simulink model "monitor"  (R2019b)
settings: Solver=FixedStepAuto  StartTime=0.0  StopTime=inf  FixedStep=0.01  RelTol=1e-3
undefined symbols (not defined in the file or in its folder): Command, f, serial
libraries: instrumentlib x5, simulink x3
settings Model: EnablePacing=on  Creator=Quinn  LastModifiedBy=Quinn

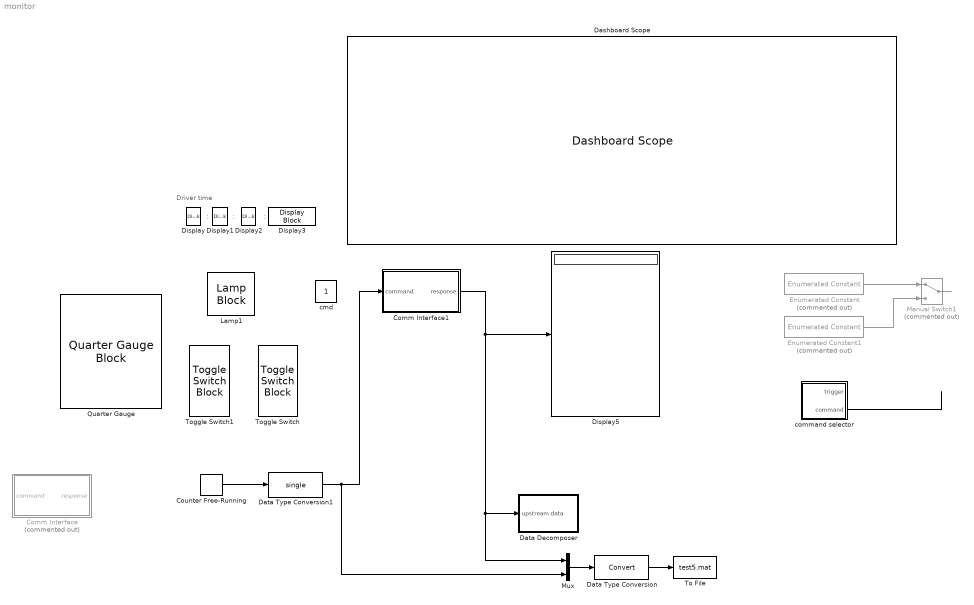
== system monitor ==
  note: :
  note: Driver time
  note: :
  note: :
  Comm Interface : Subsystem  Commented=on
  Comm Interface1 : Subsystem
  Counter Free-Running : simulink/Sources/Counter Free-Running  NumBits=16  tsamp=-1
  Dashboard Scope : DashboardScope  TimeSpan=30  Ymin=-0.5  Ymax=130
  Data Decomposer : Subsystem
  Data Type Conversion : DataTypeConversion
  Data Type Conversion1 : DataTypeConversion  OutDataTypeStr=single
  Display{,1..3} (4 alike) : DisplayBlock  LabelPosition=Hide  Format=short  Transparency=1  Opacity=0
  Display5 : Display
  Enumerated Constant : simulink/Sources/Enumerated Constant  Commented=on  OutDataTypeStr=Enum: Command  Value=Command.BX  SampleTime=inf
      settings: SourceProductName=Simulink
  Enumerated Constant1 : simulink/Sources/Enumerated Constant  Commented=on  OutDataTypeStr=Enum: Command  Value=Command.STOP  SampleTime=inf
      settings: SourceProductName=Simulink
  Lamp1 : LampBlock  LabelPosition=Bottom
  Manual Switch1 : ManualSwitch  Commented=on
  Mux : Mux  Inputs=2
  Quarter Gauge : QuarterGaugeBlock  ScaleMax=5
  To File : ToFile  Filename=test5.mat  MatrixName=data
  Toggle Switch : ToggleSwitchBlock  LabelPosition=Hide
      settings: Values={{'Log OFF', 'Log ON'}, [0 1]}
  Toggle Switch1 : ToggleSwitchBlock  LabelPosition=Hide
      settings: Values={{'PWR OFF', 'PWR ON'}, [0 1]}
  cmd : Constant  OutDataTypeStr=single
  command selector : Subsystem
  wires:
  Enumerated Constant/1 -> Manual Switch1/1
  Manual Switch1/1 -> ?
  Enumerated Constant1/1 -> Manual Switch1/2
  command selector/2(command) -> ?
  Comm Interface1/1(response) -> Mux/1, Data Decomposer/1(upstream data), Display5/1
  Data Type Conversion/1 -> To File/1
  Counter Free-Running/1 -> Data Type Conversion1/1
  Data Type Conversion1/1 -> Mux/2, Comm Interface1/1(command)
  Mux/1 -> Data Type Conversion/1

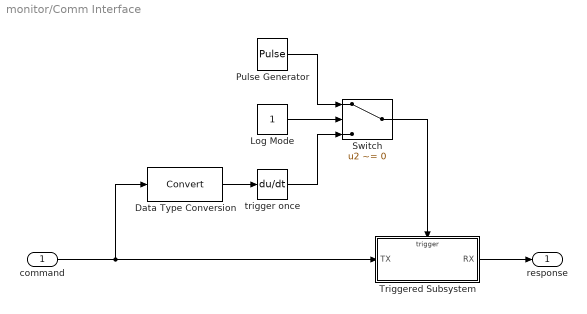
== system monitor/Comm Interface ==
  command : Inport
  Data Type Conversion : DataTypeConversion
  Log Mode : Constant
  Pulse Generator : DiscretePulseGenerator  SampleTime=0.01
  Switch : Switch  Criteria=u2 ~= 0
  Triggered Subsystem : Subsystem  Priority=1  TreatAsAtomicUnit=on
  trigger once : Derivative
  response : Outport
  wires:
  Triggered Subsystem/1(RX) -> response/1
  Log Mode/1 -> Switch/2
  Switch/1 -> Triggered Subsystem/Trigger
  Pulse Generator/1 -> Switch/1
  command/1 -> Triggered Subsystem/1(TX), Data Type Conversion/1
  trigger once/1 -> Switch/3
  Data Type Conversion/1 -> trigger once/1

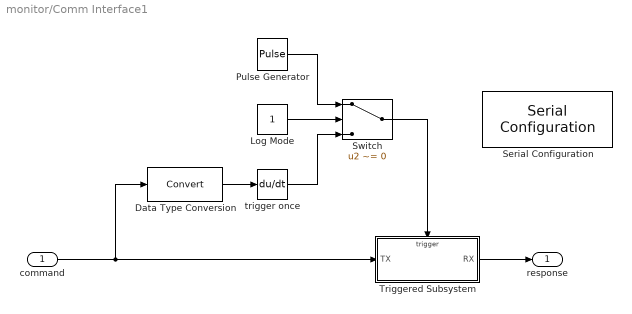
== system monitor/Comm Interface1 ==
  command : Inport
  Data Type Conversion : DataTypeConversion
  Log Mode : Constant
  Pulse Generator : DiscretePulseGenerator  SampleTime=0.01
  Serial Configuration : instrumentlib/Serial Configuration  Priority=-200000  ComPortMenu=COM5  ComPort=COM5  ObjConstructor=serial('COM5');  BaudRate=5e6  DataBits=8  Parity=none  StopBits=1  FlowControl=none  Timeout=1  ByteOrder=LittleEndian
  Switch : Switch  Criteria=u2 ~= 0
  Triggered Subsystem : Subsystem  Priority=1  TreatAsAtomicUnit=on
  trigger once : Derivative
  response : Outport
  wires:
  Data Type Conversion/1 -> trigger once/1
  trigger once/1 -> Switch/3
  command/1 -> Data Type Conversion/1, Triggered Subsystem/1(TX)
  Pulse Generator/1 -> Switch/1
  Switch/1 -> Triggered Subsystem/Trigger
  Log Mode/1 -> Switch/2
  Triggered Subsystem/1(RX) -> response/1

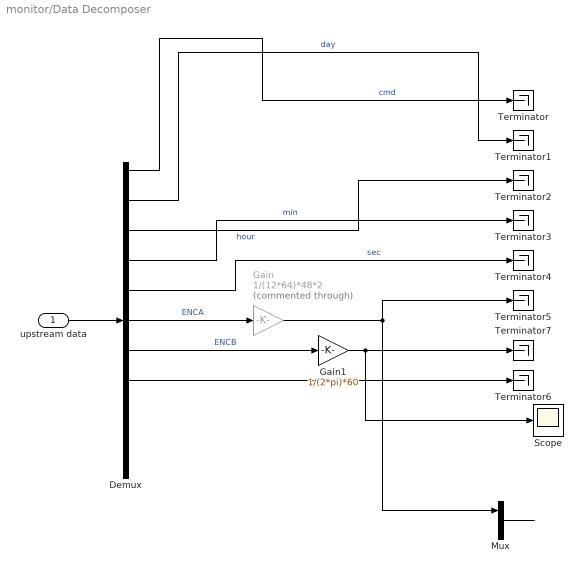
== system monitor/Data Decomposer ==
  upstream data : Inport
  Demux : Demux  Outputs=11
  Gain : Gain  Commented=through  Gain=1/(12*64)*48*2
  Gain1 : Gain  Gain=1/(2*pi)*60
  Mux : Mux  Inputs=2
  Scope : Scope
  Terminator{,1..7} (8 alike) : Terminator
  wires:
  upstream data/1 -> Demux/1
  Demux/1 -> Terminator/1  "cmd"
  Demux/3 -> Terminator2/1  "hour"
  Demux/2 -> Terminator1/1  "day"
  Demux/4 -> Terminator3/1  "min"
  Demux/5 -> Terminator4/1  "sec"
  Demux/6 -> Gain/1  "ENCA"
  Demux/8 -> Terminator6/1
  Gain/1 -> Mux/1, Terminator5/1
  Demux/7 -> Gain1/1  "ENCB"
  Gain1/1 -> Scope/1, Terminator7/1
  Mux/1 -> ?

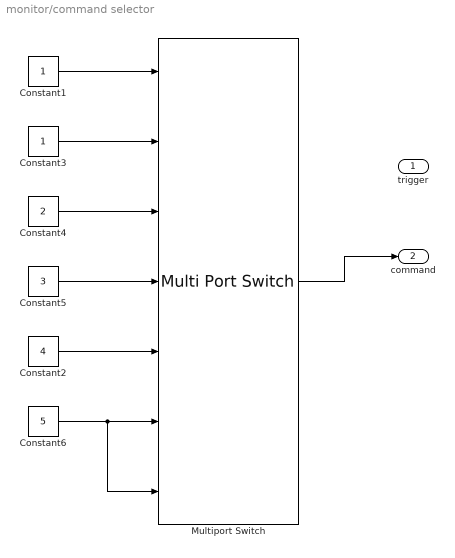
== system monitor/command selector ==
  Constant1 : Constant
  Constant2 : Constant  Value=4
  Constant3 : Constant
  Constant4 : Constant  Value=2
  Constant5 : Constant  Value=3
  Constant6 : Constant  Value=5
  Multiport Switch : MultiPortSwitch  Inputs=5  DataPortIndices={Command.INIT,Command.BX,Command.STOP}  DataPortForDefault=Additional data port  DiagnosticForDefault=Warning
  trigger : Outport
  command : Outport  Port=2
  wires:
  Constant1/1 -> Multiport Switch/1
  Constant5/1 -> Multiport Switch/4
  Constant3/1 -> Multiport Switch/2
  Constant4/1 -> Multiport Switch/3
  Multiport Switch/1 -> command/1
  Constant2/1 -> Multiport Switch/5
  Constant6/1 -> Multiport Switch/7, Multiport Switch/6

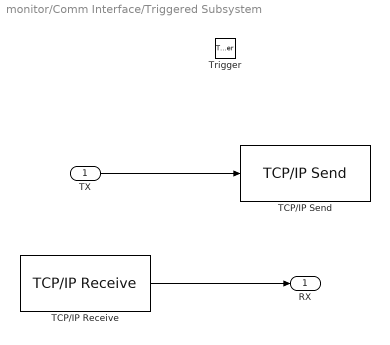
== system monitor/Comm Interface/Triggered Subsystem ==
  TX : Inport
  Trigger : TriggerPort  VariantControl=Variant
  TCP/IP Receive : instrumentlib/TCP//IP Receive  Priority=10  Host=192.168.0.7  Port=23  DataSize="[7  1]"  EnableBlockingMode=on  Timeout=3  SampleTime=-1  DataType=single  ByteOrder=LittleEndian  ASCIIFormatting=%f,  Terminator=LF
      settings: SourceProductName=Instrument Control Toolbox
  TCP/IP Send : instrumentlib/TCP//IP Send  Priority=1  Host=192.168.0.7  Port=23  EnableBlockingMode=on  Timeout=3  ByteOrder=LittleEndian  TransferDelay=on
      settings: SourceProductName=Instrument Control Toolbox
  RX : Outport
  wires:
  TCP/IP Receive/1 -> RX/1
  TX/1 -> TCP/IP Send/1

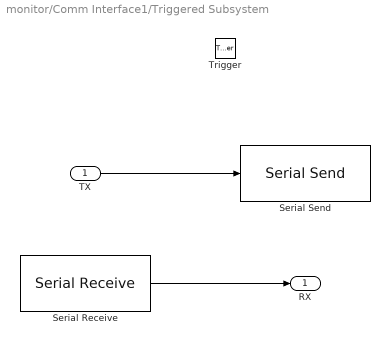
== system monitor/Comm Interface1/Triggered Subsystem ==
  TX : Inport
  Trigger : TriggerPort  TriggerType=either  VariantControl=Variant
  Serial Receive : instrumentlib/Serial Receive  Priority=10  ComPortMenu=COM5  ComPort=COM5  ObjConstructor=serial('COM5');  Terminator=<none>  DataSize="[19   1]"  DataType=single  EnableBlockingMode=on  ActionDataUnavailable=Output custom value  CustomValue=repmat(-1, 1, 19)  SampleTime=-1
  Serial Send : instrumentlib/Serial Send  Priority=1  ComPortMenu=COM5  ComPort=COM5  ObjConstructor=serial('COM5');  Terminator=<none>  EnableBlockingMode=off
  RX : Outport
  wires:
  TX/1 -> Serial Send/1
  Serial Receive/1 -> RX/1
